simulink model "Non_Linear_Quadrotor_Control"  (R2025a)
settings: Solver=VariableStepAuto  StartTime=0.0  StopTime=100  RelTol=1e-3
libraries: simulink x4, motor_propeller_Dynamics_Model x4, altitude_PD__controller x1, Horizontal_Position_Controller x1
settings Model: Creator=patri  LastModifiedBy=patri

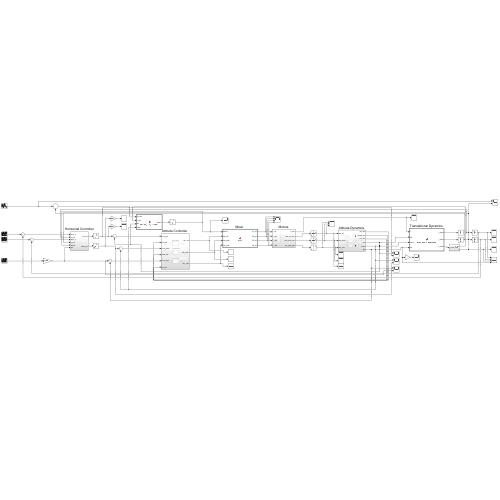
[thumbnail: Simulink's stored preview of the top-level diagram]
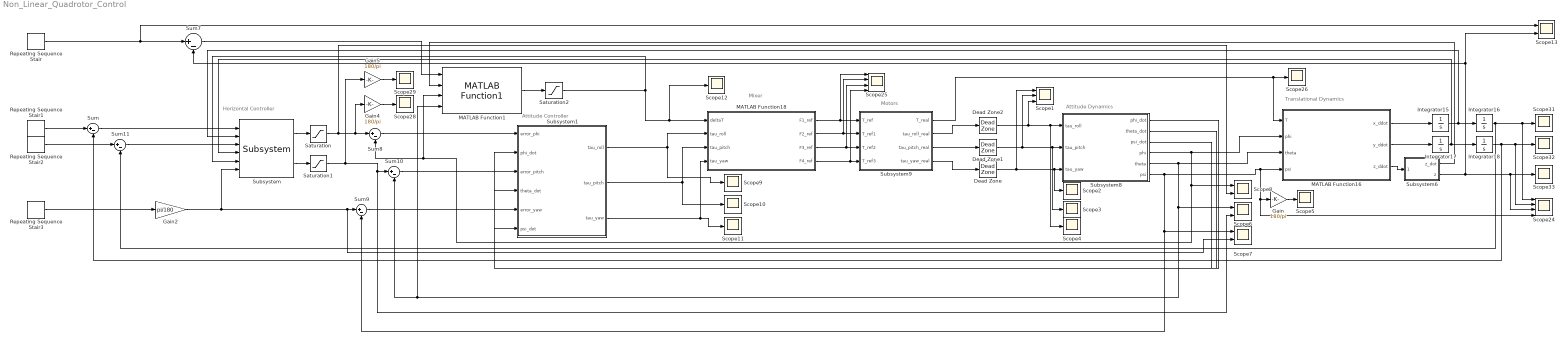
== system Non_Linear_Quadrotor_Control ==
  note: Horizontal Controller
  note: Attitude Controller
  note: Motors
  note: Attitude Dynamics
  note: Mixer
  note: Translational Dynamics
  Dead Zone : DeadZone  LowerValue=-1e-5  UpperValue=1e-5
  Dead Zone1 : DeadZone  LowerValue=-1e-5  UpperValue=1e-5
  Dead Zone2 : DeadZone  LowerValue=-1e-5  UpperValue=1e-5
  Gain : Gain  Gain=180/pi
  Gain2 : Gain  Gain=pi/180
  Gain4 : Gain  Gain=180/pi
  Gain5 : Gain  Gain=180/pi
  Integrator{15..18} (4 alike) : Integrator
  MATLAB Function1 : altitude_PD__controller/MATLAB Function1  SystemSampleTime=-1  VariantActivationTime=update diagram  EmptyChoice=off  PassThrough=off  PassThroughVariantControl=(default)  EmptyChoiceVariantControl=(default)  AllowFlexibleInterface=on  Latency=0  AutoFrameSizeCalculation=off
  MATLAB Function16 : MATLAB Function  TreatAsAtomicUnit=on
  MATLAB Function18 : MATLAB Function  TreatAsAtomicUnit=on
  Repeating Sequence Stair : simulink/Sources/Repeating Sequence Stair  OutValues=[3 1 4 2 1]  tsamp=20  OutMin=[]  OutMax=[]  OutDataTypeStr=double  OutputDataTypeScalingMode=double  OutDataType=fixdt(0,8)  ConRadixGroup=Best Precision: Vector-wise  OutScaling=2^-12
  Repeating Sequence Stair1 : simulink/Sources/Repeating Sequence Stair  OutValues=[0 3 1 2 4 3 1 2 4 3 1 2 4]  tsamp=20  OutMin=[]  OutMax=[]  OutDataTypeStr=double  OutputDataTypeScalingMode=double  OutDataType=fixdt(0,8)  ConRadixGroup=Best Precision: Vector-wise  OutScaling=2^-12
  Repeating Sequence Stair2 : simulink/Sources/Repeating Sequence Stair  OutValues=[0 1 4 2 1 1 4 2 1 1 4 2 1]  tsamp=20  OutMin=[]  OutMax=[]  OutDataTypeStr=double  OutputDataTypeScalingMode=double  OutDataType=fixdt(0,8)  ConRadixGroup=Best Precision: Vector-wise  OutScaling=2^-12
  Repeating Sequence Stair3 : simulink/Sources/Repeating Sequence Stair  OutValues=[0 10 50 90 130 10 50 90 130 10 50 90 130]  tsamp=10  OutMin=[]  OutMax=[]  OutDataTypeStr=double  OutputDataTypeScalingMode=double  OutDataType=fixdt(0,8)  ConRadixGroup=Best Precision: Vector-wise  OutScaling=2^-12
  Saturation : Saturate  UpperLimit=0.3491  LowerLimit=-0.3491
  Saturation1 : Saturate  UpperLimit=0.3491  LowerLimit=-0.3491
  Saturation2 : Saturate  UpperLimit=24.525  LowerLimit=-6.715
  Scope1 : Scope  NumInputPorts=3
      settings: ActiveDisplayYMinimum=-1  ActiveDisplayYMaximum=1
  Scope{2..5,9..12,26,28..29,31..33} (14 alike) : Scope
      Scope10 settings: ActiveDisplayYMinimum=-1  ActiveDisplayYMaximum=1  DataLoggingVariableName=ScopeData24
      Scope11 settings: ActiveDisplayYMinimum=-0.18633521823298424  ActiveDisplayYMaximum=0.17701696409685838  DataLoggingVariableName=ScopeData25
      Scope12 settings: ActiveDisplayYMinimum=-1  ActiveDisplayYMaximum=1  DataLoggingVariableName=ScopeData26
      Scope2 settings: ActiveDisplayYMinimum=-1  ActiveDisplayYMaximum=1
      Scope26 settings: ActiveDisplayYMinimum=-1  ActiveDisplayYMaximum=1  DataLoggingVariableName=ScopeData53
      Scope28 settings: ActiveDisplayYMinimum=-1  ActiveDisplayYMaximum=1  DataLoggingVariableName=ScopeData55
      Scope29 settings: ActiveDisplayYMinimum=-1  ActiveDisplayYMaximum=1  DataLoggingVariableName=ScopeData56
      Scope3 settings: ActiveDisplayYMinimum=-0.023062202009291377  ActiveDisplayYMaximum=0.3322193407049393  DataLoggingVariableName=ScopeData2
      Scope31 settings: ActiveDisplayYMinimum=-0.52584340641875671  ActiveDisplayYMaximum=4.732590657768811  DataLoggingVariableName=ScopeData58
      Scope32 settings: ActiveDisplayYMinimum=-0.37534512874718262  ActiveDisplayYMaximum=3.378106158724643  DataLoggingVariableName=ScopeData59
      Scope33 settings: ActiveDisplayYMinimum=-0.12545290649798821  ActiveDisplayYMaximum=1.1290761584818942  DataLoggingVariableName=ScopeData60
      Scope4 settings: ActiveDisplayYMinimum=-1  ActiveDisplayYMaximum=1  DataLoggingVariableName=ScopeData7
      Scope5 settings: ActiveDisplayYMinimum=-1  ActiveDisplayYMaximum=1  DataLoggingVariableName=ScopeData16
      Scope9 settings: ActiveDisplayYMinimum=-0.92199070853856979  ActiveDisplayYMaximum=0.2979163768471278  DataLoggingVariableName=ScopeData23
  Scope{6..8,13} (4 alike) : Scope  NumInputPorts=2
      Scope13 settings: ActiveDisplayYMinimum=-1.4495417439927372  ActiveDisplayYMaximum=4.6429514234678946  DataLoggingVariableName=ScopeData6
      Scope6 settings: ActiveDisplayYMinimum=-0.42894568627380236  ActiveDisplayYMaximum=0.36674321716098429  DataLoggingVariableName=ScopeData17
      Scope7 settings: ActiveDisplayYMinimum=-0.21816615649929114  ActiveDisplayYMaximum=1.9634954084936207  DataLoggingVariableName=ScopeData18
      Scope8 settings: ActiveDisplayYMinimum=-0.43637472843777619  ActiveDisplayYMaximum=0.436714051951327  DataLoggingVariableName=ScopeData21
  Scope24 : Scope  NumInputPorts=4
      settings: ActiveDisplayYMinimum=-0.502041526682306  ActiveDisplayYMaximum=4.5183737401407535  DataLoggingVariableName=ScopeData40
  Scope25 : Scope  NumInputPorts=4
      settings: ActiveDisplayYMinimum=-0.20484572010197288  ActiveDisplayYMaximum=10.248356935201397  DataLoggingVariableName=ScopeData41
  Subsystem : Horizontal_Position_Controller/Subsystem  SystemSampleTime=-1  VariantActivationTime=update diagram  EmptyChoice=off  PassThrough=off  PassThroughVariantControl=(default)  EmptyChoiceVariantControl=(default)  AllowFlexibleInterface=on  Latency=0  AutoFrameSizeCalculation=off
  Subsystem1 : Subsystem
  Subsystem6 : Subsystem
  Subsystem8 : Subsystem
  Subsystem9 : Subsystem
  Sum{,7..11} (6 alike) : Sum  Inputs=|+-
  wires:
  Integrator16/1 -> Scope24/1, Scope31/1, Sum11/2
  Subsystem9/4(tau_yaw_real) -> Dead Zone/1
  Dead Zone2/1 -> Scope1/3, Subsystem8/1(tau_roll), Scope4/1
  Subsystem8/3(psi_dot) -> Subsystem1/6(psi_dot)
  MATLAB Function18/1(F1_ref) -> Subsystem9/1(T_ref), Scope25/1
  Subsystem1/3(tau_yaw) -> MATLAB Function18/4(tau_yaw), Scope11/1
  Sum10/1 -> Subsystem1/3(error_pitch)
  Dead Zone/1 -> Subsystem8/3(tau_yaw), Scope2/1, Scope1/1
  Saturation/1 -> Sum8/1, Gain4/1, Scope8/2
  Subsystem6/1(z_dot) -> MATLAB Function1/2
  Subsystem6/2(z) -> Sum7/2, Scope13/2, Scope33/1, Scope24/3
  Subsystem8/4(phi) -> MATLAB Function1/3, Sum8/2, Scope8/1, MATLAB Function16/2(phi)
  Integrator15/1 -> Subsystem/2, Integrator16/1
  Gain/1 -> Scope5/1
  Saturation1/1 -> Gain5/1, Sum10/1, Scope6/2
  MATLAB Function16/1(x_ddot) -> Integrator15/1
  MATLAB Function1/1 -> Saturation2/1
  Gain2/1 -> Subsystem/6, Scope7/2, Sum9/1
  MATLAB Function16/2(y_ddot) -> Integrator17/1
  Sum9/1 -> Subsystem1/5(error_yaw)
  Subsystem8/2(theta_dot) -> Subsystem1/4(theta_dot)
  Sum8/1 -> Subsystem1/1(error_phi)
  Integrator17/1 -> Subsystem/4, Integrator18/1
  Subsystem8/6(psi) -> Scope24/4, Gain/1, MATLAB Function16/4(psi), Sum9/2, Scope7/1
  Gain5/1 -> Scope29/1
  Subsystem1/1(tau_roll) -> MATLAB Function18/2(tau_roll), Scope9/1
  MATLAB Function18/4(F4_ref) -> Subsystem9/4(T_ref3), Scope25/4
  Dead Zone1/1 -> Scope1/2, Subsystem8/2(tau_pitch), Scope3/1
  Subsystem1/2(tau_pitch) -> MATLAB Function18/3(tau_pitch), Scope10/1
  Integrator18/1 -> Scope24/2, Scope32/1, Sum/2
  Saturation2/1 -> Scope12/1, MATLAB Function18/1(deltaT), Subsystem/5
  Sum/1 -> Subsystem/1
  MATLAB Function18/2(F2_ref) -> Subsystem9/2(T_ref1), Scope25/2
  Gain4/1 -> Scope28/1
  Subsystem8/5(theta) -> Sum10/2, MATLAB Function1/4, Scope6/1, MATLAB Function16/3(theta)
  Subsystem9/2(tau_roll_real) -> Dead Zone2/1
  Subsystem9/1(T_real) -> MATLAB Function16/1(T), Scope26/1
  MATLAB Function16/3(z_ddot) -> Subsystem6/1(z_ddot_free)
  Subsystem8/1(phi_dot) -> Subsystem1/2(phi_dot)
  Subsystem9/3(tau_pitch_real) -> Dead Zone1/1
  Sum11/1 -> Subsystem/3
  Sum7/1 -> MATLAB Function1/1
  MATLAB Function18/3(F3_ref) -> Subsystem9/3(T_ref2), Scope25/3
  Subsystem/1 -> Saturation/1
  Subsystem/2 -> Saturation1/1
  Repeating Sequence Stair/1 -> Scope13/1, Sum7/1
  Repeating Sequence Stair1/1 -> Sum/1
  Repeating Sequence Stair2/1 -> Sum11/1
  Repeating Sequence Stair3/1 -> Gain2/1

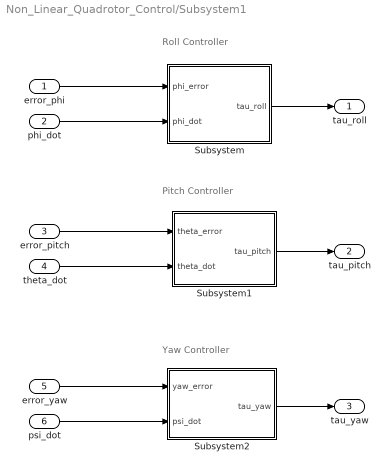
== system Non_Linear_Quadrotor_Control/Subsystem1 ==
  note: Roll Controller
  note: Pitch Controller
  note: Yaw Controller
  error_phi : Inport
  phi_dot : Inport  Port=2
  error_pitch : Inport  Port=3
  theta_dot : Inport  Port=4
  error_yaw : Inport  Port=5
  psi_dot : Inport  Port=6
  Subsystem : Subsystem
  Subsystem1 : Subsystem
  Subsystem2 : Subsystem
  tau_roll : Outport
  tau_pitch : Outport  Port=2
  tau_yaw : Outport  Port=3
  wires:
  error_phi/1 -> Subsystem/1(phi_error)
  phi_dot/1 -> Subsystem/2(phi_dot)
  Subsystem/1(tau_roll) -> tau_roll/1
  error_pitch/1 -> Subsystem1/1(theta_error)
  theta_dot/1 -> Subsystem1/2(theta_dot)
  Subsystem1/1(tau_pitch) -> tau_pitch/1
  error_yaw/1 -> Subsystem2/1(yaw_error)
  psi_dot/1 -> Subsystem2/2(psi_dot)
  Subsystem2/1(tau_yaw) -> tau_yaw/1

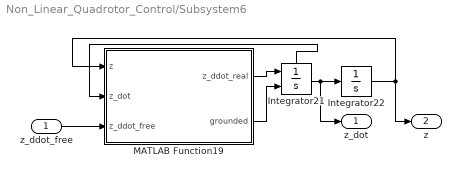
== system Non_Linear_Quadrotor_Control/Subsystem6 ==
  z_ddot_free : Inport
  Integrator21 : Integrator  ExternalReset=rising  ShowStatePort=on
  Integrator22 : Integrator  LimitOutput=on  LowerSaturationLimit=0
  MATLAB Function19 : MATLAB Function  TreatAsAtomicUnit=on
  z_dot : Outport
  z : Outport  Port=2
  wires:
  Integrator21/1 -> z_dot/1, Integrator22/1
  Integrator22/1 -> MATLAB Function19/1(z), z/1
  MATLAB Function19/1(z_ddot_real) -> Integrator21/1
  Integrator21/State -> MATLAB Function19/2(z_dot)
  MATLAB Function19/2(grounded) -> Integrator21/2
  z_ddot_free/1 -> MATLAB Function19/3(z_ddot_free)

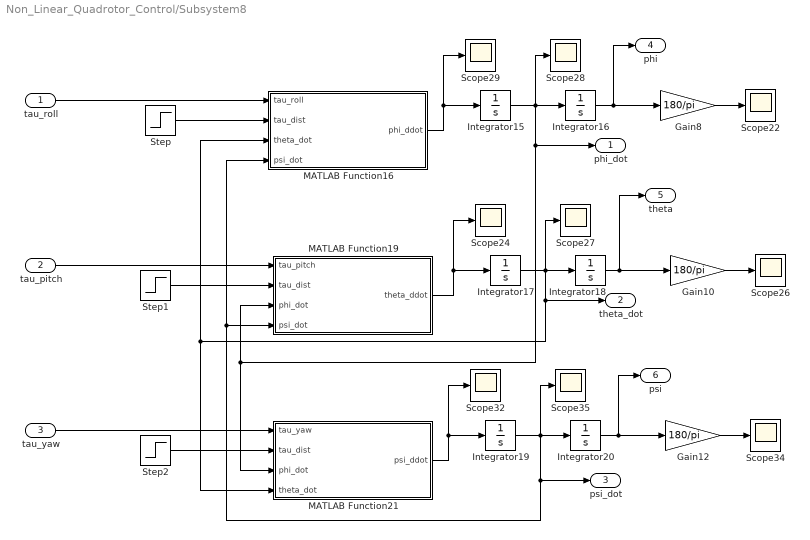
== system Non_Linear_Quadrotor_Control/Subsystem8 ==
  tau_roll : Inport
  tau_pitch : Inport  Port=2
  tau_yaw : Inport  Port=3
  Gain10 : Gain  Gain=180/pi
  Gain12 : Gain  Gain=180/pi
  Gain8 : Gain  Gain=180/pi
  Integrator{15..20} (6 alike) : Integrator
  MATLAB Function16 : MATLAB Function  TreatAsAtomicUnit=on
  MATLAB Function19 : MATLAB Function  TreatAsAtomicUnit=on
  MATLAB Function21 : MATLAB Function  TreatAsAtomicUnit=on
  Scope{22,24,26..29,32,34..35} (9 alike) : Scope
      Scope22 settings: ActiveDisplayYMinimum=-1  ActiveDisplayYMaximum=1  DataLoggingVariableName=ScopeData3
      Scope24 settings: ActiveDisplayYMinimum=-4.968236230500775  ActiveDisplayYMaximum=29.640847114405577  DataLoggingVariableName=ScopeData8
      Scope26 settings: ActiveDisplayYMinimum=-1  ActiveDisplayYMaximum=1  DataLoggingVariableName=ScopeData10
      Scope27 settings: ActiveDisplayYMinimum=-0.33682673973321314  ActiveDisplayYMaximum=1.2513613924780251  DataLoggingVariableName=ScopeData11
      Scope28 settings: ActiveDisplayYMinimum=-0.33682673973321314  ActiveDisplayYMaximum=1.2513613924780251  DataLoggingVariableName=ScopeData4
      Scope29 settings: ActiveDisplayYMinimum=-1  ActiveDisplayYMaximum=1  DataLoggingVariableName=ScopeData5
      Scope32 settings: ActiveDisplayYMinimum=-1  ActiveDisplayYMaximum=1  DataLoggingVariableName=ScopeData12
      Scope34 settings: ActiveDisplayYMinimum=-1  ActiveDisplayYMaximum=1  DataLoggingVariableName=ScopeData14
      Scope35 settings: ActiveDisplayYMinimum=-0.33682673973321314  ActiveDisplayYMaximum=1.2513613924780251  DataLoggingVariableName=ScopeData15
  Step : Step  Time=20  After=0  SampleTime=0
  Step1 : Step  Time=20  After=0  SampleTime=0
  Step2 : Step  Time=10  After=0  SampleTime=0
  phi_dot : Outport
  theta_dot : Outport  Port=2
  psi_dot : Outport  Port=3
  phi : Outport  Port=4
  theta : Outport  Port=5
  psi : Outport  Port=6
  wires:
  MATLAB Function19/1(theta_ddot) -> Scope24/1, Integrator17/1
  MATLAB Function21/1(psi_ddot) -> Scope32/1, Integrator19/1
  Gain10/1 -> Scope26/1
  Integrator16/1 -> phi/1, Gain8/1
  MATLAB Function16/1(phi_ddot) -> Scope29/1, Integrator15/1
  Gain8/1 -> Scope22/1
  Gain12/1 -> Scope34/1
  tau_pitch/1 -> MATLAB Function19/1(tau_pitch)
  tau_roll/1 -> MATLAB Function16/1(tau_roll)
  tau_yaw/1 -> MATLAB Function21/1(tau_yaw)
  Integrator18/1 -> theta/1, Gain10/1
  Integrator20/1 -> psi/1, Gain12/1
  Integrator15/1 -> Scope28/1, MATLAB Function21/3(phi_dot), MATLAB Function19/3(phi_dot), phi_dot/1, Integrator16/1
  Integrator17/1 -> MATLAB Function21/4(theta_dot), MATLAB Function16/3(theta_dot), theta_dot/1, Scope27/1, Integrator18/1
  Integrator19/1 -> MATLAB Function19/4(psi_dot), MATLAB Function16/4(psi_dot), psi_dot/1, Scope35/1, Integrator20/1
  Step/1 -> MATLAB Function16/2(tau_dist)
  Step1/1 -> MATLAB Function19/2(tau_dist)
  Step2/1 -> MATLAB Function21/2(tau_dist)

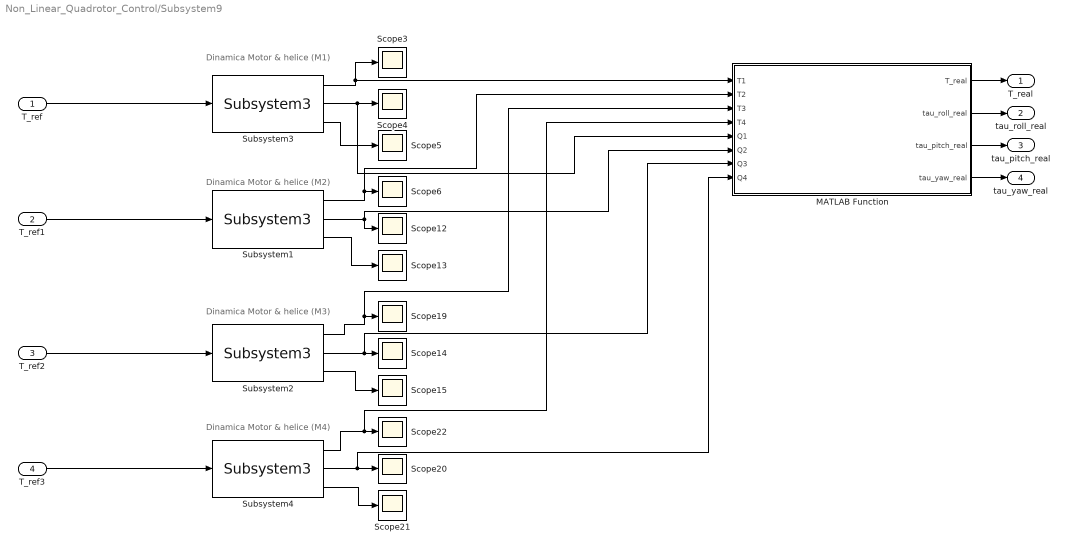
== system Non_Linear_Quadrotor_Control/Subsystem9 ==
  note: Dinamica Motor & helice (M1)
  note: Dinamica Motor & helice (M2)
  note: Dinamica Motor & helice (M3)
  note: Dinamica Motor & helice (M4)
  T_ref : Inport
  T_ref1 : Inport  Port=2
  T_ref2 : Inport  Port=3
  T_ref3 : Inport  Port=4
  MATLAB Function : MATLAB Function  TreatAsAtomicUnit=on
  Scope{3..6,12..15,19..22} (12 alike) : Scope
      Scope12 settings: ActiveDisplayYMinimum=-0.075634730162752767  ActiveDisplayYMaximum=0.0084038589069725285  DataLoggingVariableName=ScopeData28
      Scope13 settings: ActiveDisplayYMinimum=-1  ActiveDisplayYMaximum=1  DataLoggingVariableName=ScopeData29
      Scope14 settings: ActiveDisplayYMinimum=-0.075634730162752767  ActiveDisplayYMaximum=0.0084038589069725285  DataLoggingVariableName=ScopeData31
      Scope15 settings: ActiveDisplayYMinimum=-1  ActiveDisplayYMaximum=1  DataLoggingVariableName=ScopeData32
      Scope19 settings: ActiveDisplayYMinimum=-0.59524387701486947  ActiveDisplayYMaximum=5.3571948931338262  DataLoggingVariableName=ScopeData33
      Scope20 settings: ActiveDisplayYMinimum=-0.075634730162752767  ActiveDisplayYMaximum=0.0084038589069725285  DataLoggingVariableName=ScopeData34
      Scope21 settings: ActiveDisplayYMinimum=-1  ActiveDisplayYMaximum=1  DataLoggingVariableName=ScopeData35
      Scope22 settings: ActiveDisplayYMinimum=-0.80438017643413839  ActiveDisplayYMaximum=7.2394215879072474  DataLoggingVariableName=ScopeData36
      Scope3 settings: ActiveDisplayYMinimum=-0.51020554873668367  ActiveDisplayYMaximum=4.5918499386301539  DataLoggingVariableName=ScopeData19
      Scope4 settings: ActiveDisplayYMinimum=-0.075634730162752767  ActiveDisplayYMaximum=0.0084038589069725285  DataLoggingVariableName=ScopeData20
      Scope5 settings: ActiveDisplayYMinimum=-593.34405402607968  ActiveDisplayYMaximum=5340.0964862347182  DataLoggingVariableName=ScopeData27
      Scope6 settings: ActiveDisplayYMinimum=-0.7625605388924166  ActiveDisplayYMaximum=6.8630448500317511  DataLoggingVariableName=ScopeData30
  Subsystem{1..4} (4 alike) : motor_propeller_Dynamics_Model/Subsystem3  SystemSampleTime=-1  VariantActivationTime=update diagram  EmptyChoice=off  PassThrough=off  PassThroughVariantControl=(default)  EmptyChoiceVariantControl=(default)  AllowFlexibleInterface=on  Latency=0  AutoFrameSizeCalculation=off
  T_real : Outport
  tau_roll_real : Outport  Port=2
  tau_pitch_real : Outport  Port=3
  tau_yaw_real : Outport  Port=4
  wires:
  Subsystem3/3 -> Scope5/1
  Subsystem2/3 -> Scope15/1
  Subsystem1/2 -> Scope12/1, MATLAB Function/6(Q2)
  Subsystem2/2 -> Scope14/1, MATLAB Function/7(Q3)
  Subsystem4/3 -> Scope21/1
  Subsystem3/1 -> MATLAB Function/1(T1), Scope3/1
  Subsystem4/2 -> MATLAB Function/8(Q4), Scope20/1
  Subsystem2/1 -> MATLAB Function/3(T3), Scope19/1
  Subsystem3/2 -> MATLAB Function/5(Q1), Scope4/1
  T_ref2/1 -> Subsystem2/1
  Subsystem1/1 -> MATLAB Function/2(T2), Scope6/1
  Subsystem1/3 -> Scope13/1
  Subsystem4/1 -> MATLAB Function/4(T4), Scope22/1
  T_ref3/1 -> Subsystem4/1
  T_ref1/1 -> Subsystem1/1
  T_ref/1 -> Subsystem3/1
  MATLAB Function/1(T_real) -> T_real/1
  MATLAB Function/2(tau_roll_real) -> tau_roll_real/1
  MATLAB Function/3(tau_pitch_real) -> tau_pitch_real/1
  MATLAB Function/4(tau_yaw_real) -> tau_yaw_real/1

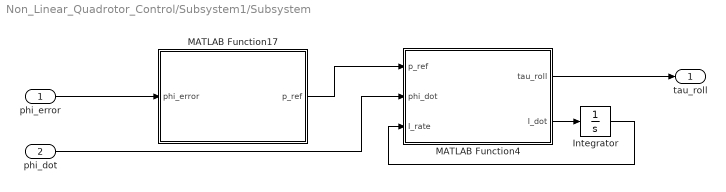
== system Non_Linear_Quadrotor_Control/Subsystem1/Subsystem ==
  phi_error : Inport
  phi_dot : Inport  Port=2
  Integrator : Integrator
  MATLAB Function17 : MATLAB Function  TreatAsAtomicUnit=on
  MATLAB Function4 : MATLAB Function  TreatAsAtomicUnit=on
  tau_roll : Outport
  wires:
  MATLAB Function17/1(p_ref) -> MATLAB Function4/1(p_ref)
  MATLAB Function4/1(tau_roll) -> tau_roll/1
  MATLAB Function4/2(I_dot) -> Integrator/1
  Integrator/1 -> MATLAB Function4/3(I_rate)
  phi_dot/1 -> MATLAB Function4/2(phi_dot)
  phi_error/1 -> MATLAB Function17/1(phi_error)

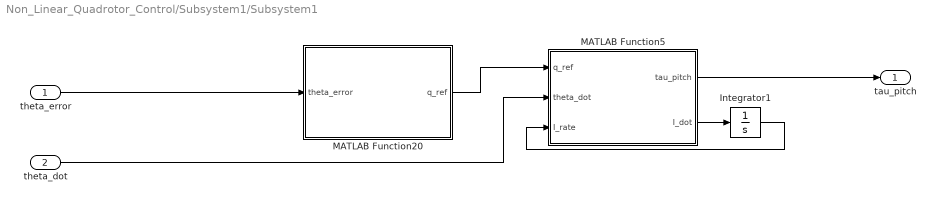
== system Non_Linear_Quadrotor_Control/Subsystem1/Subsystem1 ==
  theta_error : Inport
  theta_dot : Inport  Port=2
  Integrator1 : Integrator
  MATLAB Function20 : MATLAB Function  TreatAsAtomicUnit=on
  MATLAB Function5 : MATLAB Function  TreatAsAtomicUnit=on
  tau_pitch : Outport
  wires:
  MATLAB Function20/1(q_ref) -> MATLAB Function5/1(q_ref)
  MATLAB Function5/1(tau_pitch) -> tau_pitch/1
  Integrator1/1 -> MATLAB Function5/3(I_rate)
  theta_error/1 -> MATLAB Function20/1(theta_error)
  MATLAB Function5/2(I_dot) -> Integrator1/1
  theta_dot/1 -> MATLAB Function5/2(theta_dot)

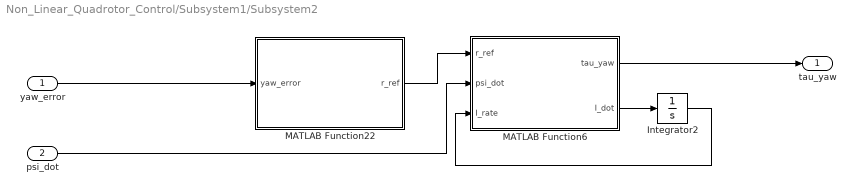
== system Non_Linear_Quadrotor_Control/Subsystem1/Subsystem2 ==
  yaw_error : Inport
  psi_dot : Inport  Port=2
  Integrator2 : Integrator
  MATLAB Function22 : MATLAB Function  TreatAsAtomicUnit=on
  MATLAB Function6 : MATLAB Function  TreatAsAtomicUnit=on
  tau_yaw : Outport
  wires:
  Integrator2/1 -> MATLAB Function6/3(I_rate)
  MATLAB Function22/1(r_ref) -> MATLAB Function6/1(r_ref)
  yaw_error/1 -> MATLAB Function22/1(yaw_error)
  psi_dot/1 -> MATLAB Function6/2(psi_dot)
  MATLAB Function6/2(I_dot) -> Integrator2/1
  MATLAB Function6/1(tau_yaw) -> tau_yaw/1

== matlab function Non_Linear_Quadrotor_Control/Subsystem8/MATLAB Function16 ==
  data: tau_roll input; phi_ddot output; tau_dist input; theta_dot input; psi_dot input
function phi_ddot = roll_dynamics( ...
    tau_roll, tau_dist, theta_dot, psi_dot)

% Provisional moments of inertia
Jx = 0.020;   % Roll  [kg.m^2]
Jy = 0.022;   % Pitch [kg.m^2]
Jz = 0.040;   % Yaw   [kg.m^2]

phi_ddot = ((Jy - Jz)/Jx)*theta_dot*psi_dot + (tau_roll + tau_dist)/Jx;

end

== matlab function Non_Linear_Quadrotor_Control/Subsystem8/MATLAB Function19 ==
  data: tau_pitch input; theta_ddot output; tau_dist input; phi_dot input; psi_dot input
function theta_ddot = pitch_dynamics( ...
    tau_pitch, tau_dist, phi_dot, psi_dot)

% Provisional moments of inertia
Jx = 0.020;   % Roll  [kg.m^2]
Jy = 0.022;   % Pitch [kg.m^2]
Jz = 0.040;   % Yaw   [kg.m^2]

theta_ddot = ((Jz - Jx)/Jy)*phi_dot*psi_dot + (tau_pitch + tau_dist)/Jy;

end

== matlab function Non_Linear_Quadrotor_Control/Subsystem8/MATLAB Function21 ==
  data: tau_yaw input; psi_ddot output; tau_dist input; phi_dot input; theta_dot input
function psi_ddot = yaw_dynamics( ...
    tau_yaw, tau_dist, phi_dot, theta_dot)

% Provisional moments of inertia
Jx = 0.020;   % Roll  [kg.m^2]
Jy = 0.022;   % Pitch [kg.m^2]
Jz = 0.040;   % Yaw   [kg.m^2]

psi_ddot = ((Jx - Jy)/Jz)*phi_dot*theta_dot + (tau_yaw + tau_dist)/Jz;

end

== matlab function Non_Linear_Quadrotor_Control/Subsystem9/MATLAB Function ==
  data: T1 input; T_real output; T2 input; T3 input; T4 input; Q1 input; Q2 input; Q3 input; Q4 input; tau_roll_real output; tau_pitch_real output; tau_yaw_real output
function [T_real, tau_roll_real, tau_pitch_real, tau_yaw_real] = ...
    calculate_forces_torques(T1, T2, T3, T4, Q1, Q2, Q3, Q4)

L = 0.2121;      % distance from center to motor
a_x = L/sqrt(2);   % effective arm for roll
a_y = L/sqrt(2);   % effective arm for pitch

T_real = T1 + T2 + T3 + T4;

tau_roll_real = a_x*(T1 - T2 - T3 + T4);

tau_pitch_real = a_y*(-T1 - T2 + T3 + T4);

tau_yaw_real = -Q1 + Q2 - Q3 + Q4;

end

== matlab function Non_Linear_Quadrotor_Control/Subsystem1/Subsystem/MATLAB Function17 ==
  data: phi_error input; p_ref output
function p_ref = roll_angle_controller(phi_error)

Kphi = 6;

p_ref = Kphi * phi_error;

% Desired angular velocity limit

p_max = 1.5; % rad/s

p_ref = min(max(p_ref,-p_max),p_max);

end

== matlab function Non_Linear_Quadrotor_Control/Subsystem1/Subsystem2/MATLAB Function6 ==
  data: r_ref input; tau_yaw output; psi_dot input; I_rate input; I_dot output
function [tau_yaw, I_dot] = yaw_rate_controller( ...
    r_ref, psi_dot, I_rate)

Kp = 0.28;%0.22
Ki = 0.25;

tau_max = 0.15; % N.m

% Angular velocity error
rate_error = r_ref - psi_dot;

% PI
tau_unsat = Kp*rate_error + Ki*I_rate;

% Saturation
tau_yaw = min(max(tau_unsat, -tau_max), tau_max);

% Anti-windup
if (tau_unsat >= tau_max && rate_error > 0) || ...
   (tau_unsat <= -tau_max && rate_error < 0)

    I_dot = 0;

else
    I_dot = rate_error;
end

end

== matlab function Non_Linear_Quadrotor_Control/Subsystem1/Subsystem1/MATLAB Function20 ==
  data: theta_error input; q_ref output
function q_ref = pitch_angle_controller(theta_error)

Ktheta = 6;

q_ref = Ktheta * theta_error;

% Desired angular velocity limit

q_max = 1.5; % rad/s

q_ref = min(max(q_ref, -q_max), q_max);

end

== matlab function Non_Linear_Quadrotor_Control/Subsystem1/Subsystem2/MATLAB Function22 ==
  data: yaw_error input; r_ref output
function r_ref = yaw_angle_controller(yaw_error)

Kpsi = 1.85;

% Keep the error between -pi and +pi

yaw_error = atan2(sin(yaw_error), cos(yaw_error));

r_ref = Kpsi * yaw_error;

% Desired angular velocity limit

r_max = 0.5; % rad/s

r_ref = min(max(r_ref, -r_max), r_max);

end

== matlab function Non_Linear_Quadrotor_Control/Subsystem1/Subsystem/MATLAB Function4 ==
  data: p_ref input; tau_roll output; phi_dot input; I_rate input; I_dot output
function [tau_roll, I_dot] = roll_rate_controller( ...
    p_ref, phi_dot, I_rate)

Kp = 0.85;
Ki = 3;

tau_max = 0.8; 

% Angular velocity error
rate_error = p_ref - phi_dot;

% PI
tau_unsat = Kp*rate_error + Ki*I_rate;

% Saturation
tau_roll = min(max(tau_unsat,-tau_max),tau_max);

% Anti-windup
if (tau_unsat >= tau_max && rate_error > 0) || ...
   (tau_unsat <= -tau_max && rate_error < 0)

    I_dot = 0;

else
    I_dot = rate_error;
end

end

== matlab function Non_Linear_Quadrotor_Control/Subsystem1/Subsystem1/MATLAB Function5 ==
  data: q_ref input; tau_pitch output; theta_dot input; I_rate input; I_dot output
function [tau_pitch, I_dot] = pitch_rate_controller( ...
    q_ref, theta_dot, I_rate)

Kp = 0.94;
Ki = 3.30;

tau_max = 0.8; % N.m

% Angular velocity error
rate_error = q_ref - theta_dot;

% PI
tau_unsat = Kp*rate_error + Ki*I_rate;

% Saturation
tau_pitch = min(max(tau_unsat, -tau_max), tau_max);

% Anti-windup
if (tau_unsat >= tau_max && rate_error > 0) || ...
   (tau_unsat <= -tau_max && rate_error < 0)

    I_dot = 0;

else
    I_dot = rate_error;
end

end

== matlab function Non_Linear_Quadrotor_Control/MATLAB Function16 ==
  data: T input; x_ddot output; phi input; theta input; psi input; y_ddot output; z_ddot output
function [x_ddot, y_ddot, z_ddot] = translational_dynamics(T, phi, theta, psi)

m = 1.5;
g = 9.81;

x_ddot = (T/m)*(cos(psi)*sin(theta)*cos(phi) + sin(psi)*sin(phi));

y_ddot = (T/m)*(sin(psi)*sin(theta)*cos(phi) - cos(psi)*sin(phi));

z_ddot = (T/m)*cos(theta)*cos(phi) - g;

end

== matlab function Non_Linear_Quadrotor_Control/MATLAB Function18 ==
  data: deltaT input; F1_ref output; tau_roll input; tau_pitch input; tau_yaw input; F2_ref output; F3_ref output; F4_ref output
function [F1_ref, F2_ref, F3_ref, F4_ref] = mixer(deltaT, tau_roll, tau_pitch, tau_yaw)

m = 1.5;
g = 9.81;

L = 0.2121;       % distance from CG
a_x = L/sqrt(2);  % effective distance for pitch
a_y = L/sqrt(2);  % effective distance for roll

d = 0.02; % Kq/kf

Fmin = 1.5;    % minimum margin during yaw maneuver [N]
Fmax = 9.81;   % maximum thrust per motor [N] - provisional

T = m*g + deltaT;

R = tau_roll / a_y;
P = tau_pitch / a_x;

% Desired yaw command
Y_cmd = -tau_yaw/d;

% Mixer without considering yaw
b1 = T + R - P;
b2 = T - R - P;
b3 = T - R + P;
b4 = T + R + P;

% Yaw limits to maintain:
% Fmin <= Fi <= Fmax

Ymin = max([b1 - 4*Fmax, ...
            4*Fmin - b2, ...
            b3 - 4*Fmax, ...
            4*Fmin - b4]);

Ymax = min([b1 - 4*Fmin, ...
            4*Fmax - b2, ...
            b3 - 4*Fmin, ...
            4*Fmax - b4]);

% Yaw saturation
Y = min(max(Y_cmd, Ymin), Ymax);

% Mixer
F1_ref = (b1 - Y)/4;
F2_ref = (b2 + Y)/4;
F3_ref = (b3 - Y)/4;
F4_ref = (b4 + Y)/4;

% Absolute physical motor limits
F1_ref = min(max(F1_ref,0),Fmax);
F2_ref = min(max(F2_ref,0),Fmax);
F3_ref = min(max(F3_ref,0),Fmax);
F4_ref = min(max(F4_ref,0),Fmax);

end

== matlab function Non_Linear_Quadrotor_Control/Subsystem6/MATLAB Function19 ==
  data: z input; z_ddot_real output; z_dot input; z_ddot_free input; grounded output
function [z_ddot_real, grounded] = contato_solo(z, z_dot, z_ddot_free)

eps_z = 1e-4;

grounded = (z <= eps_z) && (z_dot <= 0) && (z_ddot_free <= 0);

if grounded
    z_ddot_real = 0;
else
    z_ddot_real = z_ddot_free;
end

end
